simulink model "Disturbance"  (R2020b)
settings: Solver=VariableStepAuto  StartTime=0.0  StopTime=10  RelTol=1e-3
undefined symbols (not defined in the file): A, B, C, K_trackink_1, K_trackink_2
libraries: dspsrcs4 x2
settings Model: Creator=YSN  LastModifiedBy=YSN

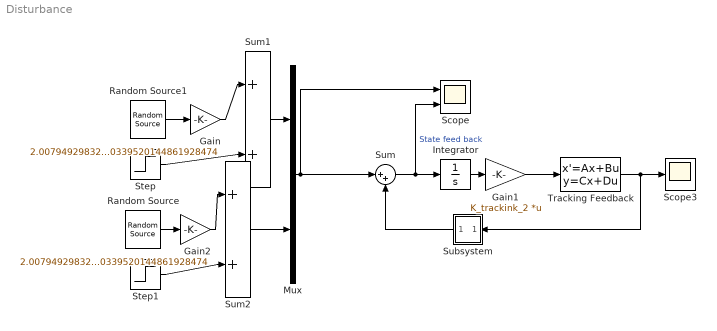
== system Disturbance ==
  Gain : Gain  Gain=2.0079492983250339520144861928474
  Gain1 : Gain  Gain=K_trackink_2  Multiplication=Matrix(K*u)
  Gain2 : Gain  Gain=2.0079492983250339520144861928474
  Integrator : Integrator
  Mux : Mux  Inputs=2
  Random Source : dspsrcs4/Random Source  SrcType=Uniform  NormMethod=Ziggurat  CltLength=12  MinVal=0  MaxVal=1  MeanVal=0  VarVal=1  RepMode=Not repeatable  rawSeed=1  IsInherit=off  SampMode=Discrete  SampTime=0.1  SampFrame=1  DataType=Double  OutComplex=Real  OutputFrames=off
  Random Source1 : dspsrcs4/Random Source  SrcType=Uniform  NormMethod=Ziggurat  CltLength=12  MinVal=0  MaxVal=1  MeanVal=0  VarVal=1  RepMode=Not repeatable  rawSeed=1  IsInherit=off  SampMode=Continuous  SampTime=0.01  SampFrame=1  DataType=Double  OutComplex=Real  OutputFrames=off
  Scope : Scope  NumInputPorts=2
  Scope3 : Scope
  Step : Step  Time=0.1  SampleTime=0
  Step1 : Step  Time=0.1  SampleTime=0
  Subsystem : Subsystem
  Sum : Sum  Inputs=|++
  Sum1 : Sum  Inputs=|++
  Sum2 : Sum  Inputs=|++
  Tracking Feedback : StateSpace  A=A-B*K_trackink_1  B=B  C=C  D=[0 0;0 0;0 0]  InitialCondition=[0 0.0 0.0 0 0 0]  ContinuousStateAttributes='Helicopter'
  wires:
  Mux/1 -> Scope/1, Sum/1
  Tracking Feedback/1 -> Subsystem/1(In1), Scope3/1
  Integrator/1 -> Gain1/1
  Sum/1 -> Scope/2, Integrator/1  "State feed back"
  Gain1/1 -> Tracking Feedback/1
  Sum1/1 -> Mux/1
  Step/1 -> Sum1/2
  Sum2/1 -> Mux/2
  Step1/1 -> Sum2/2
  Gain/1 -> Sum1/1
  Random Source1/1 -> Gain/1
  Gain2/1 -> Sum2/1
  Random Source/1 -> Gain2/1
  Subsystem/1(Out1) -> Sum/2

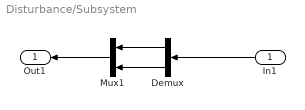
== system Disturbance/Subsystem ==
  In1 : Inport
  Demux : Demux  Outputs=3
  Mux1 : Mux  Inputs=2
  Out1 : Outport
  wires:
  Demux/1 -> Mux1/1
  Mux1/1 -> Out1/1
  Demux/3 -> Mux1/2
  In1/1 -> Demux/1
